simulink model "model"  (R2023b)
settings: Solver=ode1  StartTime=0.0  StopTime=t_final  FixedStep=0.01  RelTol=1e-3
values from neighbouring files (symbols this model uses):
  L = 0.1175    [FLC.m]    (also in calculaMatrizesModelo.m = constantes(2); ddmr_flc.m = 0; ddmr_model.m = 0)
  R = 0.034    [FLC.m]    (also in calculaMatrizesModelo.m = constantes(1); ddmr_flc.m = 0; ddmr_model.m = 0)
settings Model: Creator=Gabriel Sousa  LastModifiedBy=Gabriel Sousa
settings DebuggingCC: UnderSpecifiedDimensionMsg=warning
settings RTWCC: BuildConfiguration=Faster Runs

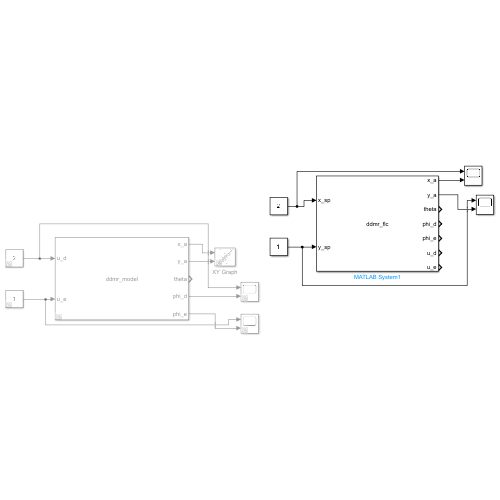
[thumbnail: Simulink's stored preview of the top-level diagram]
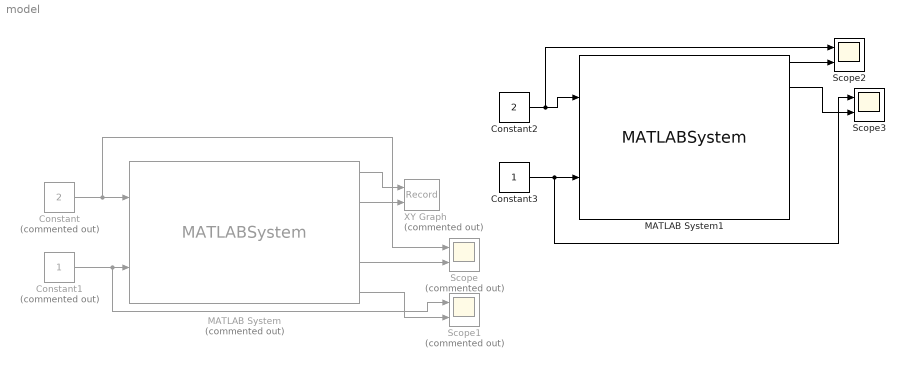
== system model ==
  Constant : Constant  Commented=on  Value=2
  Constant1 : Constant  Commented=on
  Constant2 : Constant  Value=2
  Constant3 : Constant
  MATLAB System : MATLABSystem  Commented=on  System=ddmr_model  R=R  L=L  alpha_s=alpha_s  alpha_k=alpha_k  f_s=f_s  f_k=f_k  V=V  A_tau=A_tau  B_tau=B_tau  M_i=M_i  k_i=k_i  k_p=k_p  T=0.01  SimulateUsing=Interpreted execution
      mask Type: ddmr_model
      mask Display:
      | disp('ddmr_model');
      | port_label('input',1,'u_d');
      | port_label('input',2,'u_e');
      | port_label('output',1,'x_a');
      | port_label('output',2,'y_a');
      | port_label('output',3,'theta');
      | port_label('output',4,'phi_d');
      | port_label('output',5,'phi_e');
  MATLAB System1 : MATLABSystem  System=ddmr_flc  R=R  L=L  alpha_s=alpha_s  alpha_k=alpha_k  f_s=f_s  f_k=f_k  V=V  A_tau=A_tau  B_tau=B_tau  M_i=M_i  k_i=k_i  k_p=k_p  T=0.01  fis_params=[0.066218, 0.079945, 0.4796, 0.06798, 0.84621]  SimulateUsing=Interpreted execution
      mask Type: ddmr_flc
      mask Display:
      | disp('ddmr_flc');
      | port_label('input',1,'x_sp');
      | port_label('input',2,'y_sp');
      | port_label('output',1,'x_a');
      | port_label('output',2,'y_a');
      | port_label('output',3,'theta');
      | port_label('output',4,'phi_d');
      | port_label('output',5,'phi_e');
      | port_label('output',6,'u_d');
      | port_label('output',7,'u_e');
  Scope : Scope  Commented=on  NumInputPorts=2
  Scope1 : Scope  Commented=on  NumInputPorts=2
  Scope2 : Scope  NumInputPorts=2
  Scope3 : Scope  NumInputPorts=2
  XY Graph : Record  Commented=on  FileSettingsInternal="{\"entries\":[{\"content\":{\"excelSettings\":{\"content\":{},\"type\":\"Streamout.ExcelSettings\"}},\"type\":\"Streamout.FileSettingStorage\",\"uuid\":\"\"}],\"packageUris\":[\"http:\\/\\/schema.mathworks.com\\/mf0\\/streamout_blocks\\/R2020a\"],\"version\":\"1.0\"}"  Layout=[1 1]  SignalsInternal="{\"entries\":[{\"content\":{\"signals\":[{\"content\":{\"blockPath\":[],\"dimensions\":[1,1],\"domain\":\"\",\"lineColor\":\"#a2142f\",\"plots\":[1],\"port\":1,\"sid\":[\"\"],\"signalID\":2074,\"signalName\":\"MATLAB System:1\"},\"type\":\"RecordBlkView.Signal\",\"uuid\":\"\"},{\"content\":{\"blockPath\":[],\"dimensions\":[1,1],\"domain\":\"\",\"lineColor\":\"#139fff\",\"plots\":[1],\"port\":2,\"sid\":[\"\"],\"signalID\":2078,\"signalName\":\"MATLAB System:2\"},\"type\":\"RecordBlkView.Signal\",\"uuid\":\"\"}]},\"type\":\"RecordBlkView.InputSignals\",\"uuid\":\"\"}],\"packageUris\":[\"http:\\/\\/schema.mathworks.com\\/mf0\\/streamout_blocks\\/R2020a\"],\"version\":\"1.0\"}"  VisualizationBindings="{\"xyplotplugin\":{\"info\":[{\"series\":[{\"bindingParametersList\":[{\"parameter\":\"X-Axis\",\"signalID\":2074,\"signalName\":\"MATLAB System:1\"},{\"parameter\":\"Y-Axis\",\"signalID\":2078,\"signalName\":\"MATLAB System:2\"}],\"seriesID\":10028}],\"subplotID\":1}]}}"  CompatibilityTag=XY
  wires:
  Constant/1 -> Scope/1, MATLAB System/1
  Constant1/1 -> Scope1/1, MATLAB System/2
  MATLAB System/1 -> XY Graph/1
  MATLAB System/2 -> XY Graph/2
  MATLAB System/4 -> Scope/2
  MATLAB System/5 -> Scope1/2
  Constant2/1 -> Scope2/1, MATLAB System1/1
  Constant3/1 -> Scope3/1, MATLAB System1/2
  MATLAB System1/1 -> Scope2/2
  MATLAB System1/2 -> Scope3/2
